simulink model "BionicBaroreflex"  (Simulink 7.5)
settings: Solver=ode45  StartTime=0.0  StopTime=3600  RelTol=1e-3
undefined symbols (not defined in the file or in its folder): get
libraries: simulink x11, dspstat3 x4, dspsnks4 x2, dspbuff3 x2, dspspect3 x2
settings Model: Creator=admin  LastModifiedBy=Peidro
settings DebuggingCC: StrictBusMsg=Warning

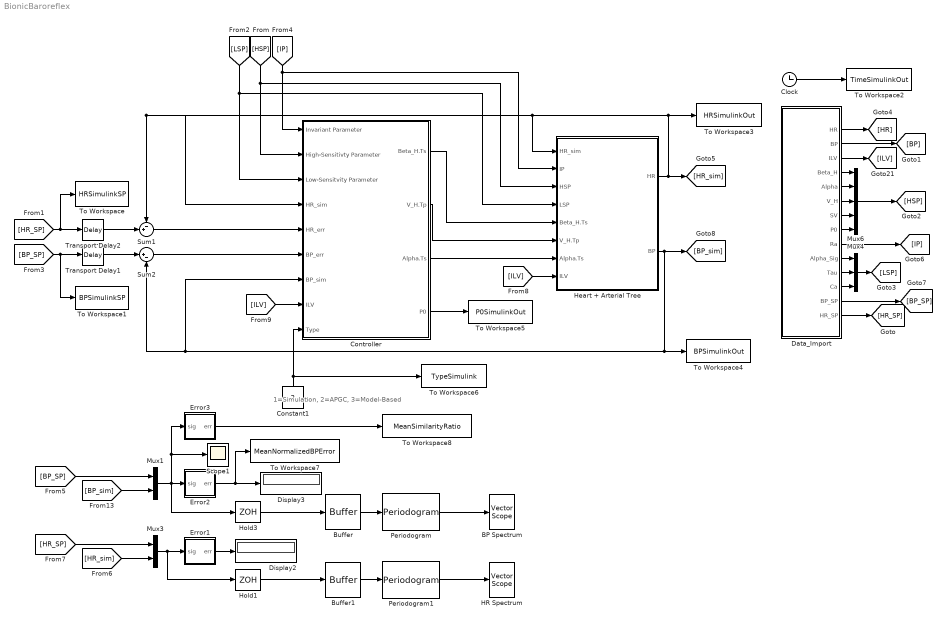
== system BionicBaroreflex ==
  note: 1=Simulation,
      | 2=APGC,
      | 3=Model-Based
  BP Spectrum : dspsnks4/Vector Scope  DialogController=dspdialog.VectorScope  DialogControllerArgs=DataTag0  ScopeProperties=on  Domain=Frequency  HorizSpan=1  DisplayProperties=off  AxisGrid=on  Memory=on  FrameNumber=on  AxisLegend=on  AxisZoom=off  OpenScopeAtSimStart=on  OpenScopeImmediately=off  FigPos=get(0,'defaultfigureposition')  AxisProperties=off  XUnits=Hertz  XRange=[0...Fs/2]  InheritXIncr=off  XIncr=1  XLabel=Time  XLimit=Auto  XMin=0  XMax=0.5  XStart=0  YUnits=dB  YLabel=Amplitude  LineProperties=off  LineColors=[1 0 0]|[0 0 1]  XAxisParamsVer=6.9
      settings: YMin=-106.7264  YMax=8.3849
  Buffer : dspbuff3/Buffer  N=128  V=64  ic=0
  Buffer1 : dspbuff3/Buffer  N=128  V=64  ic=0
  Clock : Clock
      settings: Decimation=10
  Constant1 : Constant  Value=2  OutDataType=fixdt(1, 16)  OutScaling=2^0
  Controller : Subsystem
  Data_Import : Subsystem
  Display2 : Display
  Display3 : Display
  Error1 : Subsystem
  Error2 : Subsystem
  Error3 : Subsystem
  HR Spectrum : dspsnks4/Vector Scope  DialogController=dspdialog.VectorScope  DialogControllerArgs=DataTag5  ScopeProperties=on  Domain=Frequency  HorizSpan=1  DisplayProperties=off  AxisGrid=on  Memory=on  FrameNumber=on  AxisLegend=on  AxisZoom=off  OpenScopeAtSimStart=on  OpenScopeImmediately=off  FigPos=get(0,'defaultfigureposition')  AxisProperties=off  XUnits=Hertz  XRange=[0...Fs/2]  InheritXIncr=off  XIncr=1  XLabel=Time  XLimit=Auto  XMin=0  XMax=0.5  XStart=0  YUnits=dB  YLabel=Amplitude  LineProperties=off  LineColors=[1 0 0]|[0 0 1]  XAxisParamsVer=6.9
      settings: YMin=-106.7264  YMax=8.3849
  Heart + Arterial Tree : Subsystem
  Hold1 : ZeroOrderHold  SampleTime=10
  Hold3 : ZeroOrderHold  SampleTime=10
  Mux1 : Mux  Inputs=2
  Mux3 : Mux  Inputs=2
  Mux4 : Mux  Inputs=3
  Mux6 : Mux  Inputs=5
  Periodogram : dspspect3/Periodogram  SystemSampleTime=-1  measurement=Power spectral density  wintype=Hamming  Rs=50  beta=5  winsamp=Periodic  inheritFFT=off  fftsize=128  navg=2  inheritTs=on  Ts=1
  Periodogram1 : dspspect3/Periodogram  SystemSampleTime=-1  measurement=Power spectral density  wintype=Hamming  Rs=50  beta=5  winsamp=Periodic  inheritFFT=off  fftsize=128  navg=2  inheritTs=on  Ts=1
  Scope1 : Scope
      settings: YMin=67.5  YMax=125
  Sum1 : Sum  Inputs=-+|  OutDataType=fixdt(1, 16)  OutScaling=2^0
  Sum2 : Sum  Inputs=|+-  OutDataType=fixdt(1, 16)  OutScaling=2^0
  To Workspace : ToWorkspace  VariableName=HRSimulinkSP  SampleTime=-1  SaveFormat=Structure
  To Workspace1 : ToWorkspace  VariableName=BPSimulinkSP  SampleTime=-1  SaveFormat=Structure
  To Workspace2 : ToWorkspace  VariableName=TimeSimulinkOut  SampleTime=-1  SaveFormat=Structure
  To Workspace3 : ToWorkspace  VariableName=HRSimulinkOut  SampleTime=-1  SaveFormat=Structure
  To Workspace4 : ToWorkspace  VariableName=BPSimulinkOut  SampleTime=-1  SaveFormat=Structure
  To Workspace5 : ToWorkspace  VariableName=P0SimulinkOut  SampleTime=-1  SaveFormat=Structure
  To Workspace6 : ToWorkspace  VariableName=TypeSimulink  SampleTime=-1  SaveFormat=Structure
  To Workspace7 : ToWorkspace  VariableName=MeanNormalizedBPError  SampleTime=-1  SaveFormat=Structure
  To Workspace8 : ToWorkspace  VariableName=MeanSimilarityRatio  SampleTime=-1  SaveFormat=Structure
  Transport Delay1 : TransportDelay  DelayTime=10
  Transport Delay2 : TransportDelay  DelayTime=10
  wires:
  Data_Import/1(HR) -> [HR]
  [ILV] -> Controller/8(ILV)
  Heart + Arterial Tree/1(HR) -> [HR_sim], To Workspace3/1, Sum1/1, Controller/4(HR_sim), Heart + Arterial Tree/1(HR_sim)
  Controller/1(Beta_H.Ts) -> Heart + Arterial Tree/5(Beta_H.Ts)
  Controller/2(V_H.Tp) -> Heart + Arterial Tree/6(V_H.Tp)
  Controller/3(Alpha.Ts) -> Heart + Arterial Tree/7(Alpha.Ts)
  Constant1/1 -> Controller/9(Type), To Workspace6/1
  Heart + Arterial Tree/2(BP) -> [BP_sim], Sum2/2, Controller/7(BP_sim), To Workspace4/1
  [BP_SP] -> To Workspace1/1, Transport Delay1/1
  [HR_SP] -> To Workspace/1, Transport Delay2/1
  [HSP] -> Controller/2(High-Sensitivty Parameter), Heart + Arterial Tree/3(HSP)
  [LSP] -> Controller/3(Low-Sensitvity Parameter), Heart + Arterial Tree/4(LSP)
  Mux6/1 -> [HSP]
  Mux4/1 -> [LSP]
  [IP] -> Controller/1(Invariant Parameter), Heart + Arterial Tree/2(IP)
  Mux1/1 -> Error2/1(sig), Hold3/1, Scope1/1, Error3/1(sig)
  Error2/1(err) -> Display3/1, To Workspace7/1
  Mux3/1 -> Error1/1(sig), Hold1/1
  Error1/1(err) -> Display2/1
  [HR_SP] -> Mux3/1
  [HR_sim] -> Mux3/2
  [BP_SP] -> Mux1/1
  Sum1/1 -> Controller/5(HR_err)
  Sum2/1 -> Controller/6(BP_err)
  Periodogram/1 -> BP Spectrum/1
  Hold3/1 -> Buffer/1
  Buffer/1 -> Periodogram/1
  [BP_sim] -> Mux1/2
  Periodogram1/1 -> HR Spectrum/1
  Hold1/1 -> Buffer1/1
  Buffer1/1 -> Periodogram1/1
  Data_Import/2(BP) -> [BP]
  Data_Import/3(ILV) -> [ILV]
  Data_Import/4(Beta_H) -> Mux6/1
  Data_Import/5(Alpha) -> Mux6/2
  Data_Import/6(V_H) -> Mux6/3
  Data_Import/7(SV) -> Mux6/4
  Data_Import/8(P0) -> Mux6/5
  Data_Import/9(Ra) -> [IP]
  Data_Import/10(Alpha_Sig) -> Mux4/1
  Data_Import/11(Tau) -> Mux4/2
  Data_Import/12(Ca) -> Mux4/3
  Data_Import/13(BP_SP) -> [BP_SP]
  Data_Import/14(HR_SP) -> [HR_SP]
  Clock/1 -> To Workspace2/1
  Controller/4(P0) -> To Workspace5/1
  [ILV] -> Heart + Arterial Tree/8(ILV)
  Transport Delay2/1 -> Sum1/2
  Transport Delay1/1 -> Sum2/1
  Error3/1(err) -> To Workspace8/1

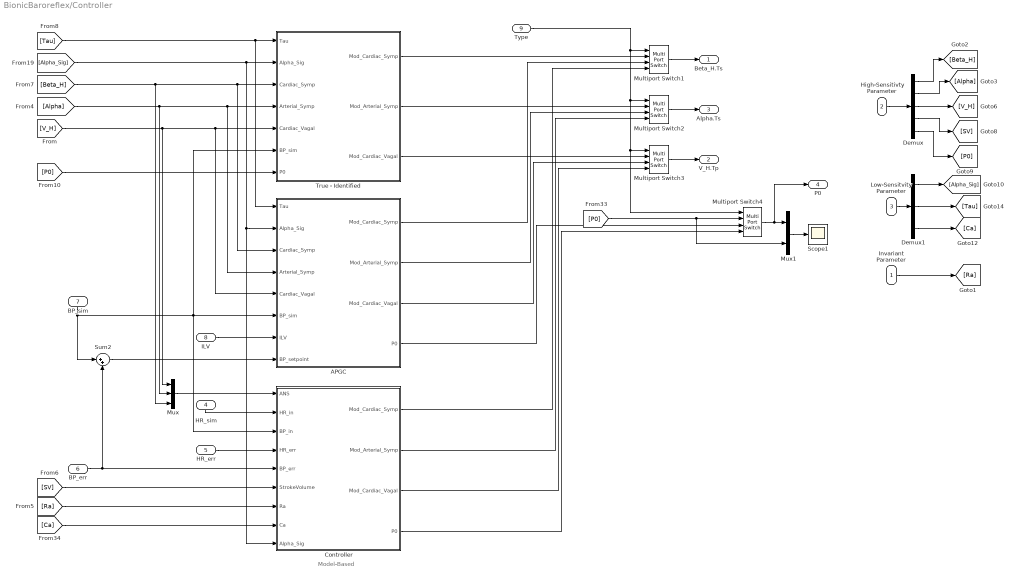
== system BionicBaroreflex/Controller ==
  note: Model-Based
  Invariant Parameter : Inport
  High-Sensitivty Parameter : Inport  Port=2
  Low-Sensitvity Parameter : Inport  Port=3
  HR_sim : Inport  Port=4
  HR_err : Inport  Port=5
  BP_err : Inport  Port=6
  BP_sim : Inport  Port=7
  ILV : Inport  Port=8
  Type : Inport  Port=9
  "APGC " : Subsystem
  Controller : Subsystem
  Demux : Demux  Outputs=5
  Demux1 : Demux  Outputs=3
  Multiport Switch{1..4} (4 alike) : MultiPortSwitch  zeroidx=off  OutDataType=fixdt(1, 16)  OutScaling=2^0
  Mux : Mux  Inputs=3
  Mux1 : Mux  Inputs=2
  Scope1 : Scope
      settings: YMin=1.725  YMax=1.925  SaveName=ScopeData2
  Sum2 : Sum  Inputs=|++  OutDataType=fixdt(1, 16)  OutScaling=2^0
  True - Identified : Subsystem
  Beta_H.Ts : Outport
  V_H.Tp : Outport  Port=2
  Alpha.Ts : Outport  Port=3
  P0 : Outport  Port=4
  wires:
  [Tau] -> True - Identified/1(Tau), "APGC "/1(Tau)
  [Beta_H] -> True - Identified/3(Cardiac_Symp), "APGC "/3(Cardiac_Symp), Mux/3
  [Alpha] -> True - Identified/4(Arterial_Symp), "APGC "/4(Arterial_Symp), Mux/2
  [V_H] -> True - Identified/5(Cardiac_Vagal), "APGC "/5(Cardiac_Vagal), Mux/1
  BP_sim/1 -> True - Identified/6(BP_sim), Controller/3(BP_in), "APGC "/6(BP_sim), Sum2/1
  [P0] -> True - Identified/7(P0)
  ILV/1 -> "APGC "/7(ILV)
  True - Identified/1(Mod_Cardiac_Symp) -> Multiport Switch1/2
  Multiport Switch1/1 -> Beta_H.Ts/1
  True - Identified/2(Mod_Arterial_Symp) -> Multiport Switch2/2
  True - Identified/3(Mod_Cardiac_Vagal) -> Multiport Switch3/2
  Controller/1(Mod_Cardiac_Symp) -> Multiport Switch1/4
  Controller/2(Mod_Arterial_Symp) -> Multiport Switch2/4
  Controller/3(Mod_Cardiac_Vagal) -> Multiport Switch3/4
  Mux/1 -> Controller/1(ANS)
  Type/1 -> Multiport Switch2/1, Multiport Switch3/1, Multiport Switch4/1, Multiport Switch1/1
  Controller/4(P0) -> Multiport Switch4/4
  [Ra] -> Controller/7(Ra)
  [Ca] -> Controller/8(Ca)
  [SV] -> Controller/6(StrokeVolume)
  HR_err/1 -> Controller/4(HR_err)
  BP_err/1 -> Sum2/2, Controller/5(BP_err)
  High-Sensitivty Parameter/1 -> Demux/1
  Demux/1 -> [Beta_H]
  Demux/2 -> [Alpha]
  Demux/3 -> [V_H]
  Demux/4 -> [SV]
  Demux/5 -> [P0]
  Low-Sensitvity Parameter/1 -> Demux1/1
  Demux1/1 -> [Alpha_Sig]
  Demux1/2 -> [Tau]
  Demux1/3 -> [Ca]
  [Alpha_Sig] -> True - Identified/2(Alpha_Sig), "APGC "/2(Alpha_Sig), Controller/9(Alpha_Sig)
  Invariant Parameter/1 -> [Ra]
  HR_sim/1 -> Controller/2(HR_in)
  Multiport Switch2/1 -> Alpha.Ts/1
  Multiport Switch3/1 -> V_H.Tp/1
  Sum2/1 -> "APGC "/8(BP_setpoint)
  [P0] -> Multiport Switch4/2, Mux1/2
  Multiport Switch4/1 -> Mux1/1, P0/1
  Mux1/1 -> Scope1/1
  "APGC "/1(Mod_Cardiac_Symp) -> Multiport Switch1/3
  "APGC "/2(Mod_Arterial_Symp) -> Multiport Switch2/3
  "APGC "/3(Mod_Cardiac_Vagal) -> Multiport Switch3/3
  "APGC "/4(P0) -> Multiport Switch4/3

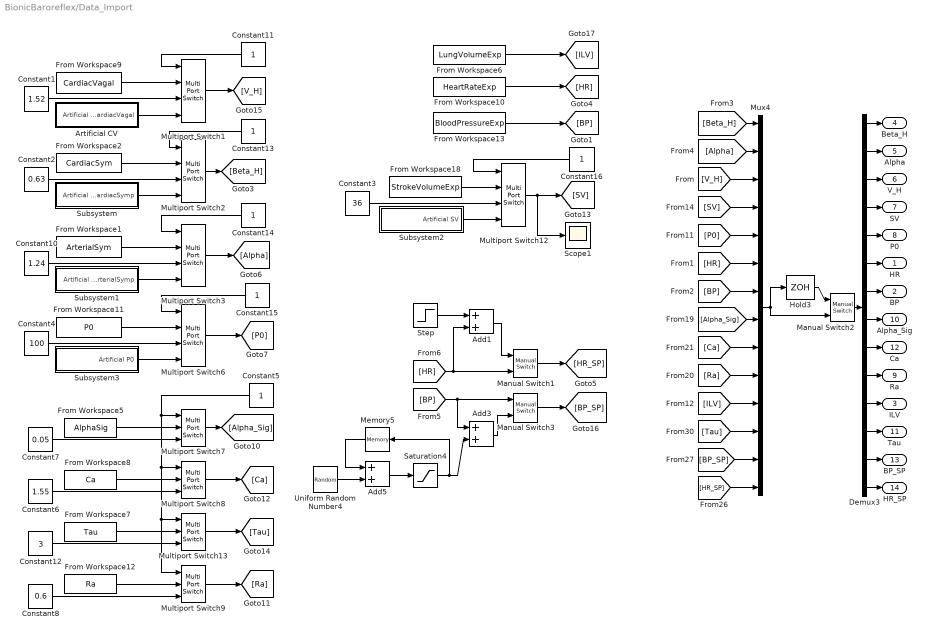
== system BionicBaroreflex/Data_Import ==
  Add1 : Sum  OutDataType=fixdt(1, 16)  OutScaling=2^-10
  Add3 : Sum  OutDataType=fixdt(1, 16)  OutScaling=2^-10
  Add5 : Sum  OutDataType=fixdt(1, 16)  OutScaling=2^-10
  Artificial CV : Subsystem
  Constant1 : Constant  Value=1.52  OutDataType=fixdt(1, 16)  OutScaling=2^0
  Constant10 : Constant  Value=1.24  OutDataType=fixdt(1, 16)  OutScaling=2^0
  Constant{5,11,13..16} (6 alike) : Constant  OutDataType=fixdt(1, 16)  OutScaling=2^0
  Constant12 : Constant  Value=3  OutDataType=fixdt(1, 16)  OutScaling=2^0
  Constant2 : Constant  Value=0.63  OutDataType=fixdt(1, 16)  OutScaling=2^0
  Constant3 : Constant  Value=36  OutDataType=fixdt(1, 16)  OutScaling=2^0
  Constant4 : Constant  Value=100  OutDataType=fixdt(1, 16)  OutScaling=2^0
  Constant6 : Constant  Value=1.55  OutDataType=fixdt(1, 16)  OutScaling=2^0
  Constant7 : Constant  Value=0.05  OutDataType=fixdt(1, 16)  OutScaling=2^0
  Constant8 : Constant  Value=0.6  OutDataType=fixdt(1, 16)  OutScaling=2^0
  Demux3 : Demux  Outputs=14
  From Workspace1 : FromWorkspace  VariableName=ArterialSym  SampleTime=1
  From Workspace10 : FromWorkspace  VariableName=HeartRateExp  SampleTime=1
  From Workspace11 : FromWorkspace  VariableName=P0  SampleTime=1
  From Workspace12 : FromWorkspace  VariableName=Ra  SampleTime=0
  From Workspace13 : FromWorkspace  VariableName=BloodPressureExp  SampleTime=1
  From Workspace18 : FromWorkspace  VariableName=StrokeVolumeExp  SampleTime=1
  From Workspace2 : FromWorkspace  VariableName=CardiacSym  SampleTime=1
  From Workspace5 : FromWorkspace  VariableName=AlphaSig  SampleTime=0
  From Workspace6 : FromWorkspace  VariableName=LungVolumeExp  SampleTime=1
  From Workspace7 : FromWorkspace  VariableName=Tau  SampleTime=0
  From Workspace8 : FromWorkspace  VariableName=Ca  SampleTime=0
  From Workspace9 : FromWorkspace  VariableName=CardiacVagal  SampleTime=1
  Hold3 : ZeroOrderHold  SampleTime=5
  Manual Switch1 : simulink/Signal Routing/Manual Switch  SystemSampleTime=-1  sw=0  action=0  varsize=off
  Manual Switch2 : simulink/Signal Routing/Manual Switch  SystemSampleTime=-1  sw=0  action=0  varsize=off
  Manual Switch3 : simulink/Signal Routing/Manual Switch  SystemSampleTime=-1  sw=1  action=0  varsize=off
  Memory5 : Memory  X0=1.3
  Multiport Switch{1..3,6,12} (5 alike) : MultiPortSwitch  zeroidx=off  OutDataType=fixdt(1, 16)  OutScaling=2^0
  Multiport Switch{7..9,13} (4 alike) : MultiPortSwitch  Inputs=2  zeroidx=off  OutDataType=fixdt(1, 16)  OutScaling=2^0
  Mux4 : Mux  Inputs=14
  Saturation4 : Saturate  UpperLimit=25  LowerLimit=-25  OutDataType=fixdt(1, 16)  OutScaling=2^0
  Scope1 : Scope
      settings: YMin=1  YMax=1.95  SaveName=ScopeData5
  Step : Step  Time=1000  SampleTime=0
  Subsystem : Subsystem
  Subsystem1 : Subsystem
  Subsystem2 : Subsystem
  Subsystem3 : Subsystem
  Uniform Random Number4 : UniformRandomNumber  Minimum=-0.1  Maximum=0.1  SampleTime=500
  HR : Outport
  BP : Outport  Port=2
  ILV : Outport  Port=3
  Beta_H : Outport  Port=4
  Alpha : Outport  Port=5
  V_H : Outport  Port=6
  SV : Outport  Port=7
  P0 : Outport  Port=8
  Ra : Outport  Port=9
  Alpha_Sig : Outport  Port=10
  Tau : Outport  Port=11
  Ca : Outport  Port=12
  BP_SP : Outport  Port=13
  HR_SP : Outport  Port=14
  wires:
  [V_H] -> Mux4/3
  [SV] -> Mux4/4
  [Alpha] -> Mux4/2
  [P0] -> Mux4/5
  [Beta_H] -> Mux4/1
  Hold3/1 -> Manual Switch2/1
  Manual Switch2/1 -> Demux3/1
  Demux3/1 -> Beta_H/1
  Demux3/3 -> V_H/1
  Demux3/2 -> Alpha/1
  Demux3/4 -> SV/1
  Demux3/5 -> P0/1
  [HR] -> Mux4/6
  [BP] -> Mux4/7
  Demux3/6 -> HR/1
  Demux3/7 -> BP/1
  [Alpha_Sig] -> Mux4/8
  Demux3/8 -> Alpha_Sig/1
  Mux4/1 -> Hold3/1, Manual Switch2/2
  [Ca] -> Mux4/9
  [Ra] -> Mux4/10
  Demux3/9 -> Ca/1
  Demux3/10 -> Ra/1
  From Workspace5/1 -> Multiport Switch7/2
  From Workspace8/1 -> Multiport Switch8/2
  From Workspace12/1 -> Multiport Switch9/2
  Multiport Switch7/1 -> [Alpha_Sig]
  Multiport Switch8/1 -> [Ca]
  Multiport Switch9/1 -> [Ra]
  Constant6/1 -> Multiport Switch8/3
  Constant7/1 -> Multiport Switch7/3
  Constant8/1 -> Multiport Switch9/3
  Constant5/1 -> Multiport Switch7/1, Multiport Switch8/1, Multiport Switch13/1, Multiport Switch9/1
  [ILV] -> Mux4/11
  Demux3/11 -> ILV/1
  From Workspace7/1 -> Multiport Switch13/2
  Multiport Switch13/1 -> [Tau]
  Constant12/1 -> Multiport Switch13/3
  [Tau] -> Mux4/12
  Demux3/12 -> Tau/1
  From Workspace10/1 -> [HR]
  From Workspace13/1 -> [BP]
  Demux3/13 -> BP_SP/1
  Demux3/14 -> HR_SP/1
  [HR_SP] -> Mux4/14
  [BP_SP] -> Mux4/13
  From Workspace6/1 -> [ILV]
  From Workspace18/1 -> Multiport Switch12/2
  Constant3/1 -> Multiport Switch12/3
  Constant16/1 -> Multiport Switch12/1
  Multiport Switch12/1 -> [SV], Scope1/1
  Multiport Switch6/1 -> [P0]
  Multiport Switch3/1 -> [Alpha]
  Multiport Switch2/1 -> [Beta_H]
  Multiport Switch1/1 -> [V_H]
  From Workspace9/1 -> Multiport Switch1/2
  From Workspace2/1 -> Multiport Switch2/2
  From Workspace1/1 -> Multiport Switch3/2
  From Workspace11/1 -> Multiport Switch6/2
  Constant1/1 -> Multiport Switch1/3
  Constant2/1 -> Multiport Switch2/3
  Constant10/1 -> Multiport Switch3/3
  Constant4/1 -> Multiport Switch6/3
  Constant11/1 -> Multiport Switch1/1
  Constant13/1 -> Multiport Switch2/1
  Constant14/1 -> Multiport Switch3/1
  Constant15/1 -> Multiport Switch6/1
  Artificial CV/1(Artificial CardiacVagal) -> Multiport Switch1/4
  Subsystem/1(Artificial CardiacSymp) -> Multiport Switch2/4
  Subsystem1/1(Artificial ArterialSymp) -> Multiport Switch3/4
  Subsystem3/1(Artificial P0) -> Multiport Switch6/4
  Subsystem2/1(Artificial SV) -> Multiport Switch12/4
  [HR] -> Manual Switch1/2, Add1/2
  Manual Switch1/1 -> [HR_SP]
  [BP] -> Manual Switch3/1, Add3/1
  Manual Switch3/1 -> [BP_SP]
  Step/1 -> Add1/1
  Add1/1 -> Manual Switch1/1
  Memory5/1 -> Add5/1
  Uniform Random Number4/1 -> Add5/2
  Add5/1 -> Saturation4/1
  Saturation4/1 -> Memory5/1, Add3/2
  Add3/1 -> Manual Switch3/2

== system BionicBaroreflex/Error1 ==
  sig : Inport
  Abs1 : Abs  OutDataType=fixdt(1, 16)  OutScaling=2^0
  Add1 : Sum  Inputs=-+  OutDataType=fixdt(1, 16)  OutScaling=2^-10
  Correlation : dspstat3/Correlation  DialogController=dspDDGCreate  DialogControllerArgs=DataTag1  domain=Time  outputDataTypeStr=Inherit: Same as accumulator  outputLastDataTypeStr=Inherit: Same as accumulator  outputMin=[]  outputMax=[]  roundingMode=Floor  overflowMode=off
  Demux : Demux  Outputs=2
  Divide : Product  Inputs=/*  OutDataType=fixdt(1, 16)  OutScaling=2^-10
  Mean : dspstat3/Mean  DialogController=dspDDGCreate  DialogControllerArgs=DataTag2  run=off  reset_popup=None  directionMode=Each column  dimension=1  treatSBRowAsCol=on  roiEnable=off  roiType=Rectangles  roiPortion=Entire ROI  roiOutput=Individual statistics for each ROI  roiFlag=off  outputDataTypeStr=Inherit: Same as accumulator  outputLastDataTypeStr=Inherit: Same as accumulator  outputMin=[]  outputMax=[]  roundingMode=Floor  overflowMode=off
  Scope : Scope
      settings: SaveName=ScopeData4
  err : Outport
  wires:
  sig/1 -> Demux/1
  Mean/1 -> err/1
  Divide/1 -> Mean/1
  Abs1/1 -> Divide/2
  Demux/2 -> Add1/2, Correlation/2
  Demux/1 -> Divide/1, Add1/1, Correlation/1
  Add1/1 -> Abs1/1
  Correlation/1 -> Scope/1

== system BionicBaroreflex/Error2 ==
  sig : Inport
  Abs1 : Abs  OutDataType=fixdt(1, 16)  OutScaling=2^0
  Add1 : Sum  Inputs=-+  OutDataType=fixdt(1, 16)  OutScaling=2^-10
  Demux : Demux  Outputs=2
  Divide : Product  Inputs=/*  OutDataType=fixdt(1, 16)  OutScaling=2^-10
  Mean : dspstat3/Mean  DialogController=dspDDGCreate  DialogControllerArgs=DataTag3  run=off  reset_popup=None  directionMode=Each column  dimension=1  treatSBRowAsCol=on  roiEnable=off  roiType=Rectangles  roiPortion=Entire ROI  roiOutput=Individual statistics for each ROI  roiFlag=off  outputDataTypeStr=Inherit: Same as accumulator  outputLastDataTypeStr=Inherit: Same as accumulator  outputMin=[]  outputMax=[]  roundingMode=Floor  overflowMode=off
  err : Outport
  wires:
  Add1/1 -> Abs1/1
  Demux/1 -> Add1/1, Divide/1
  Demux/2 -> Add1/2
  Abs1/1 -> Divide/2
  Divide/1 -> Mean/1
  Mean/1 -> err/1
  sig/1 -> Demux/1

== system BionicBaroreflex/Error3 ==
  sig : Inport
  Demux : Demux  Outputs=2
  Divide : Product  Inputs=/*  OutDataType=fixdt(1, 16)  OutScaling=2^-10
  Mean : dspstat3/Mean  DialogController=dspDDGCreate  DialogControllerArgs=DataTag4  run=off  reset_popup=None  directionMode=Each column  dimension=1  treatSBRowAsCol=on  roiEnable=off  roiType=Rectangles  roiPortion=Entire ROI  roiOutput=Individual statistics for each ROI  roiFlag=off  outputDataTypeStr=Inherit: Same as accumulator  outputLastDataTypeStr=Inherit: Same as accumulator  outputMin=[]  outputMax=[]  roundingMode=Floor  overflowMode=off
  err : Outport
  wires:
  sig/1 -> Demux/1
  Mean/1 -> err/1
  Divide/1 -> Mean/1
  Demux/2 -> Divide/2
  Demux/1 -> Divide/1

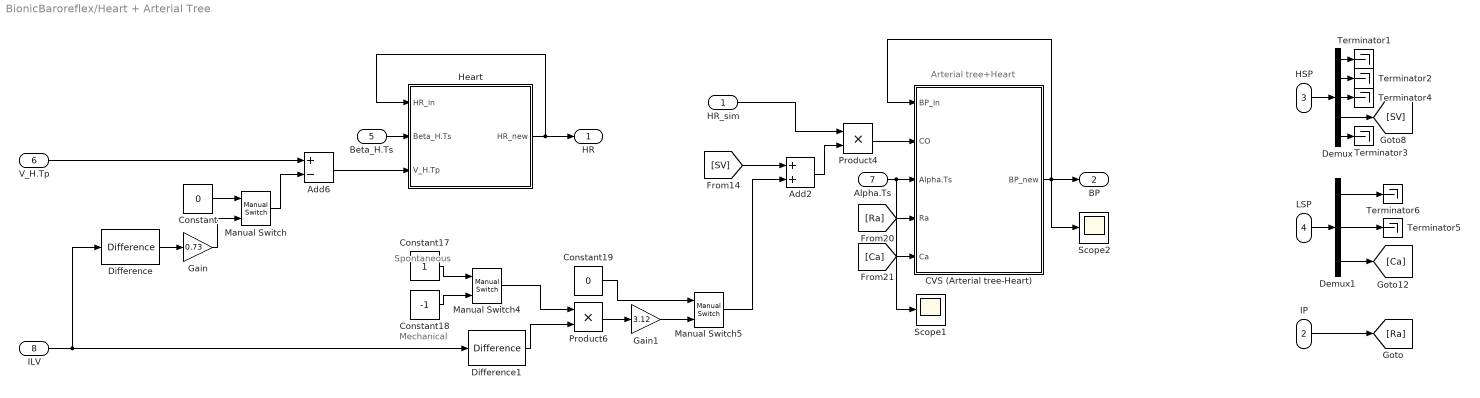
== system BionicBaroreflex/Heart + Arterial Tree ==
  note: Arterial tree+Heart
  note: Mechanical
  note: Spontaneous
  HR_sim : Inport
  IP : Inport  Port=2
  HSP : Inport  Port=3
  LSP : Inport  Port=4
  Beta_H.Ts : Inport  Port=5
  V_H.Tp : Inport  Port=6
  Alpha.Ts : Inport  Port=7
  ILV : Inport  Port=8
  Add2 : Sum  OutDataType=fixdt(1, 16)  OutScaling=2^-10
  Add6 : Sum  Inputs=+-  OutDataType=fixdt(1, 16)  OutScaling=2^-10
  CVS (Arterial tree-Heart) : Subsystem
  Constant : Constant  Value=0  OutDataType=fixdt(1, 16)  OutScaling=2^0
  Constant17 : Constant  OutDataType=fixdt(1, 16)  OutScaling=2^0
  Constant18 : Constant  Value=-1  OutDataType=fixdt(1, 16)  OutScaling=2^0
  Constant19 : Constant  Value=0  OutDataType=fixdt(1, 16)  OutScaling=2^0
  Demux : Demux  Outputs=5
  Demux1 : Demux  Outputs=3
  Difference : simulink/Discrete/Difference  SystemSampleTime=-1  ICPrevInput=0.0  OutMin=[]  OutMax=[]  OutDataType=fixdt(1, 16)  OutScaling=2^-10  DoSatur=off
  Difference1 : simulink/Discrete/Difference  SystemSampleTime=-1  ICPrevInput=0.0  OutMin=[]  OutMax=[]  OutDataType=fixdt(1, 16)  OutScaling=2^-10  DoSatur=off
  Gain : Gain  Gain=0.73  ParameterDataType=fixdt(1, 16)  ParameterScaling=2^0  OutDataType=fixdt(1, 16)  OutScaling=2^0
  Gain1 : Gain  Gain=3.12  ParameterDataType=fixdt(1, 16)  ParameterScaling=2^0  OutDataType=fixdt(1, 16)  OutScaling=2^0
  Heart : Subsystem
  Manual Switch : simulink/Signal Routing/Manual Switch  SystemSampleTime=-1  sw=1  action=0  varsize=off
  Manual Switch4 : simulink/Signal Routing/Manual Switch  SystemSampleTime=-1  sw=1  action=0  varsize=off
  Manual Switch5 : simulink/Signal Routing/Manual Switch  SystemSampleTime=-1  sw=1  action=0  varsize=off
  Product4 : Product  OutDataType=fixdt(1, 16)  OutScaling=2^0  RndMeth=Zero
  Product6 : Product  OutDataType=fixdt(1, 16)  OutScaling=2^0  RndMeth=Zero
  Scope1 : Scope
      settings: YMin=-1500  YMax=1250  SaveName=ScopeData11
  Scope2 : Scope
      settings: YMin=-1500  YMax=1250
  Terminator{1..6} (6 alike) : Terminator
  HR : Outport
  BP : Outport  Port=2
  wires:
  CVS (Arterial tree-Heart)/1(BP_new) -> CVS (Arterial tree-Heart)/1(BP_in), BP/1, Scope2/1
  Heart/1(HR_new) -> Heart/1(HR_in), HR/1
  [Ra] -> CVS (Arterial tree-Heart)/4(Ra)
  [Ca] -> CVS (Arterial tree-Heart)/5(Ca)
  Beta_H.Ts/1 -> Heart/2(Beta_H.Ts)
  Alpha.Ts/1 -> CVS (Arterial tree-Heart)/3(Alpha.Ts), Scope1/1
  LSP/1 -> Demux1/1
  Demux1/1 -> Terminator6/1
  Demux1/2 -> Terminator5/1
  Demux1/3 -> [Ca]
  IP/1 -> [Ra]
  HSP/1 -> Demux/1
  Demux/1 -> Terminator1/1
  Demux/2 -> Terminator2/1
  Demux/3 -> Terminator4/1
  Demux/4 -> [SV]
  Demux/5 -> Terminator3/1
  Product4/1 -> CVS (Arterial tree-Heart)/2(CO)
  Constant17/1 -> Manual Switch4/1
  Constant18/1 -> Manual Switch4/2
  Manual Switch4/1 -> Product6/1
  Difference1/1 -> Product6/2
  Product6/1 -> Gain1/1
  Manual Switch5/1 -> Add2/2
  Constant19/1 -> Manual Switch5/1
  ILV/1 -> Difference1/1, Difference/1
  Gain1/1 -> Manual Switch5/2
  HR_sim/1 -> Product4/1
  [SV] -> Add2/1
  Add2/1 -> Product4/2
  Gain/1 -> Manual Switch/2
  Constant/1 -> Manual Switch/1
  Difference/1 -> Gain/1
  Add6/1 -> Heart/3(V_H.Tp)
  V_H.Tp/1 -> Add6/1
  Manual Switch/1 -> Add6/2

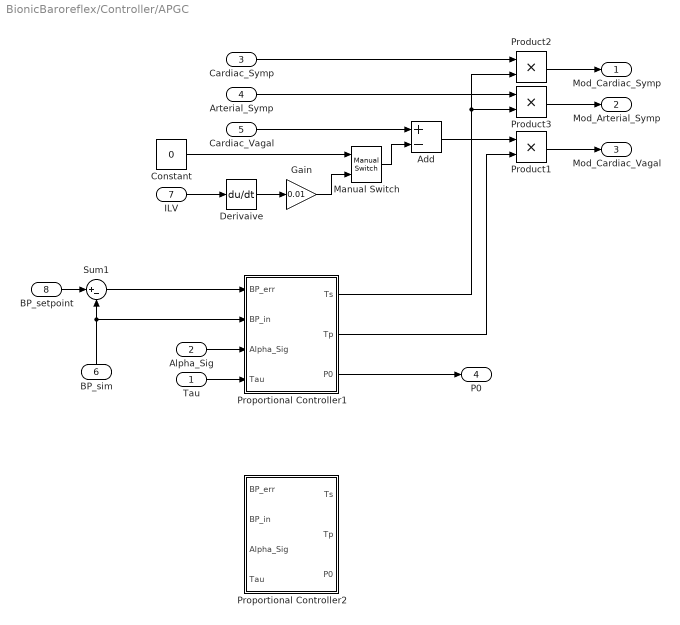
== system BionicBaroreflex/Controller/APGC  ==
  Tau : Inport
  Alpha_Sig : Inport  Port=2
  Cardiac_Symp : Inport  Port=3
  Arterial_Symp : Inport  Port=4
  Cardiac_Vagal : Inport  Port=5
  BP_sim : Inport  Port=6
  ILV : Inport  Port=7
  BP_setpoint : Inport  Port=8
  Add : Sum  Inputs=+-  OutDataType=fixdt(1, 16)  OutScaling=2^-10
  Constant : Constant  Value=0  OutDataType=fixdt(1, 16)  OutScaling=2^0
  Derivaive : Derivative
  Gain : Gain  Gain=0.01  ParameterDataType=fixdt(1, 16)  ParameterScaling=2^0  OutDataType=fixdt(1, 16)  OutScaling=2^0
  Manual Switch : simulink/Signal Routing/Manual Switch  SystemSampleTime=-1  sw=1  action=0  varsize=off
  Product1 : Product  OutDataType=fixdt(1, 16)  OutScaling=2^0  RndMeth=Zero
  Product2 : Product  OutDataType=fixdt(1, 16)  OutScaling=2^0  RndMeth=Zero
  Product3 : Product  OutDataType=fixdt(1, 16)  OutScaling=2^0  RndMeth=Zero
  Proportional Controller1 : Subsystem
  Proportional Controller2 : Subsystem
  Sum1 : Sum  Inputs=|+-  OutDataType=fixdt(1, 16)  OutScaling=2^0
  Mod_Cardiac_Symp : Outport
  Mod_Arterial_Symp : Outport  Port=2
  Mod_Cardiac_Vagal : Outport  Port=3
  P0 : Outport  Port=4
  wires:
  Cardiac_Symp/1 -> Product2/1
  Product2/1 -> Mod_Cardiac_Symp/1
  Arterial_Symp/1 -> Product3/1
  Product3/1 -> Mod_Arterial_Symp/1
  Product1/1 -> Mod_Cardiac_Vagal/1
  Add/1 -> Product1/1
  Cardiac_Vagal/1 -> Add/1
  ILV/1 -> Derivaive/1
  Derivaive/1 -> Gain/1
  Gain/1 -> Manual Switch/2
  Manual Switch/1 -> Add/2
  Constant/1 -> Manual Switch/1
  Proportional Controller1/3(P0) -> P0/1
  Proportional Controller1/2(Tp) -> Product1/2
  Proportional Controller1/1(Ts) -> Product3/2, Product2/2
  BP_setpoint/1 -> Sum1/1
  Sum1/1 -> Proportional Controller1/1(BP_err)
  Alpha_Sig/1 -> Proportional Controller1/3(Alpha_Sig)
  Tau/1 -> Proportional Controller1/4(Tau)
  BP_sim/1 -> Sum1/2, Proportional Controller1/2(BP_in)

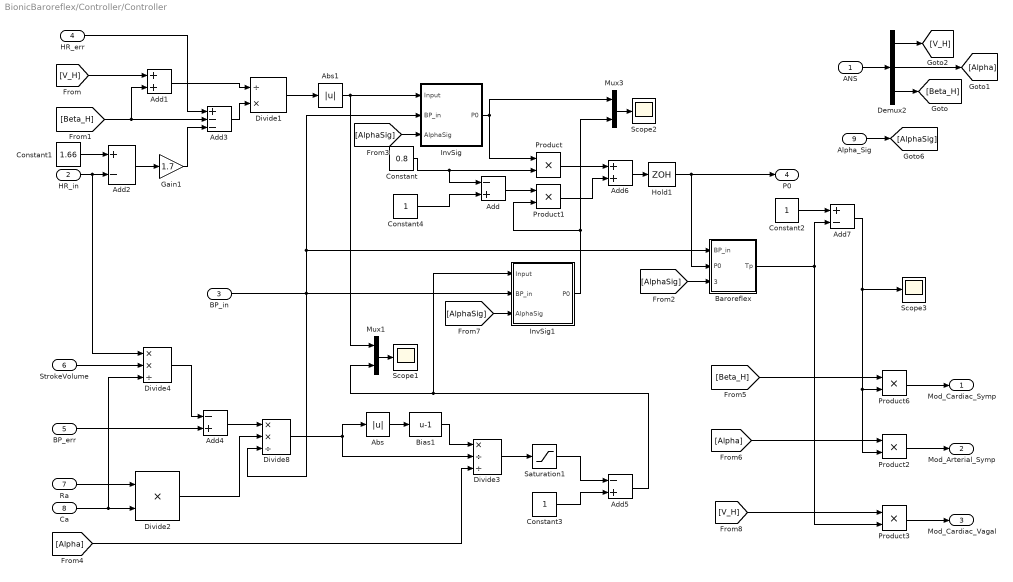
== system BionicBaroreflex/Controller/Controller ==
  ANS : Inport
  HR_in : Inport  Port=2
  BP_in : Inport  Port=3
  HR_err : Inport  Port=4
  BP_err : Inport  Port=5
  StrokeVolume : Inport  Port=6
  Ra : Inport  Port=7
  Ca : Inport  Port=8
  Alpha_Sig : Inport  Port=9
  Abs : Abs  OutDataType=fixdt(1, 16)  OutScaling=2^0
  Abs1 : Abs  OutDataType=fixdt(1, 16)  OutScaling=2^0
  Add : Sum  Inputs=-+  OutDataType=fixdt(1, 16)  OutScaling=2^-10
  Add1 : Sum  OutDataType=fixdt(1, 16)  OutScaling=2^-10
  Add2 : Sum  Inputs=+-  OutDataType=fixdt(1, 16)  OutScaling=2^-10
  Add3 : Sum  Inputs=+--  OutDataType=fixdt(1, 16)  OutScaling=2^-10
  Add4 : Sum  Inputs=-+  OutDataType=fixdt(1, 16)  OutScaling=2^-10
  Add5 : Sum  Inputs=-+  OutDataType=fixdt(1, 16)  OutScaling=2^-10
  Add6 : Sum  OutDataType=fixdt(1, 16)  OutScaling=2^-10
  Add7 : Sum  Inputs=+-  OutDataType=fixdt(1, 16)  OutScaling=2^-10
  Baroreflex : Subsystem
  Bias1 : Bias  Bias=-1
  Constant : Constant  Value=0.8  OutDataType=fixdt(1, 16)  OutScaling=2^0
  Constant1 : Constant  Value=1.66  OutDataType=fixdt(1, 16)  OutScaling=2^0
  Constant2 : Constant  OutDataType=fixdt(1, 16)  OutScaling=2^0
  Constant3 : Constant  OutDataType=fixdt(1, 16)  OutScaling=2^0
  Constant4 : Constant  OutDataType=fixdt(1, 16)  OutScaling=2^0
  Demux2 : Demux  Outputs=3
  Divide1 : Product  Inputs=/*  OutDataType=fixdt(1, 16)  OutScaling=2^-10
  Divide2 : Product  Inputs=**  OutDataType=fixdt(1, 16)  OutScaling=2^-10
  Divide3 : Product  Inputs=*//  OutDataType=fixdt(1, 16)  OutScaling=2^-10
  Divide4 : Product  Inputs=**/  OutDataType=fixdt(1, 16)  OutScaling=2^-10
  Divide8 : Product  Inputs=**/  OutDataType=fixdt(1, 16)  OutScaling=2^-10
  Gain1 : Gain  Gain=1.7  ParameterDataType=fixdt(1, 16)  ParameterScaling=2^0  OutDataType=fixdt(1, 16)  OutScaling=2^0
  Hold1 : ZeroOrderHold  SampleTime=10
  InvSig : Subsystem
  InvSig1 : Subsystem
  Mux1 : Mux  Inputs=2
  Mux3 : Mux  Inputs=2
  Product{,1..3,6} (5 alike) : Product  OutDataType=fixdt(1, 16)  OutScaling=2^0  RndMeth=Zero
  Saturation1 : Saturate  UpperLimit=1  LowerLimit=0  OutDataType=fixdt(1, 16)  OutScaling=2^0
  Scope1 : Scope
      settings: YMin=-13  YMax=1  SaveName=ScopeData18
  Scope2 : Scope
      settings: YMin=90  YMax=230  SaveName=ScopeData21
  Scope3 : Scope
      settings: YMin=90  YMax=230  SaveName=ScopeData22
  Mod_Cardiac_Symp : Outport
  Mod_Arterial_Symp : Outport  Port=2
  Mod_Cardiac_Vagal : Outport  Port=3
  P0 : Outport  Port=4
  wires:
  BP_err/1 -> Add4/2
  HR_err/1 -> Add3/1
  HR_in/1 -> Add2/2, Divide4/1
  Constant1/1 -> Add2/1
  Add3/1 -> Divide1/2
  Add1/1 -> Divide1/1
  Gain1/1 -> Add3/3
  Add2/1 -> Gain1/1
  [Beta_H] -> Add3/2, Add1/2
  [V_H] -> Add1/1
  BP_in/1 -> InvSig1/2(BP_in), Divide8/3, InvSig/2(BP_in), Baroreflex/1(BP_in)
  InvSig/1(P0) -> Mux3/1, Product/1
  Divide2/1 -> Divide8/2
  Divide8/1 -> Divide3/2, Abs/1
  Add4/1 -> Divide8/1
  Ca/1 -> Divide4/3, Divide2/2
  Ra/1 -> Divide2/1
  Divide4/1 -> Add4/1
  InvSig1/1(P0) -> Mux3/2, Product1/2
  Mux3/1 -> Scope2/1
  Mux1/1 -> Scope1/1
  Abs/1 -> Bias1/1
  Bias1/1 -> Divide3/1
  [Alpha] -> Divide3/3
  Divide3/1 -> Saturation1/1
  Constant3/1 -> Add5/2
  Add5/1 -> InvSig1/1(Input), Mux1/2
  Saturation1/1 -> Add5/1
  Add6/1 -> Hold1/1
  Baroreflex/1(Tp) -> Product3/2, Add7/2
  Constant2/1 -> Add7/1
  [AlphaSig] -> InvSig1/3(AlphaSig)
  [AlphaSig] -> InvSig/3(AlphaSig)
  [AlphaSig] -> Baroreflex/3(Alpha_Sig)
  Add7/1 -> Product2/2, Product6/2, Scope3/1
  Product/1 -> Add6/1
  ANS/1 -> Demux2/1
  Demux2/2 -> [Alpha]
  Divide1/1 -> Abs1/1
  Demux2/3 -> [Beta_H]
  Demux2/1 -> [V_H]
  Abs1/1 -> Mux1/1, InvSig/1(Input)
  Constant/1 -> Product/2, Add/1
  Product1/1 -> Add6/2
  Add/1 -> Product1/1
  Constant4/1 -> Add/2
  StrokeVolume/1 -> Divide4/2
  Alpha_Sig/1 -> [AlphaSig]
  Hold1/1 -> P0/1, Baroreflex/2(P0)
  [Beta_H] -> Product6/1
  Product6/1 -> Mod_Cardiac_Symp/1
  [Alpha] -> Product2/1
  Product2/1 -> Mod_Arterial_Symp/1
  [V_H] -> Product3/1
  Product3/1 -> Mod_Cardiac_Vagal/1

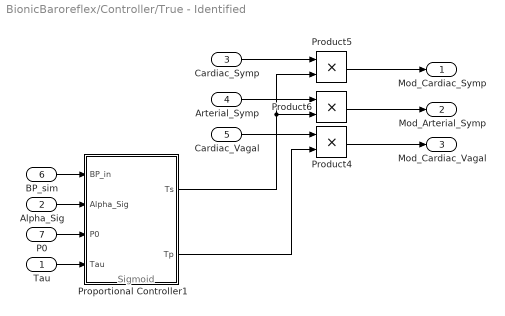
== system BionicBaroreflex/Controller/True - Identified ==
  note: Sigmoid
  Tau : Inport
  Alpha_Sig : Inport  Port=2
  Cardiac_Symp : Inport  Port=3
  Arterial_Symp : Inport  Port=4
  Cardiac_Vagal : Inport  Port=5
  BP_sim : Inport  Port=6
  P0 : Inport  Port=7
  Product4 : Product  OutDataType=fixdt(1, 16)  OutScaling=2^0  RndMeth=Zero
  Product5 : Product  OutDataType=fixdt(1, 16)  OutScaling=2^0  RndMeth=Zero
  Product6 : Product  OutDataType=fixdt(1, 16)  OutScaling=2^0  RndMeth=Zero
  Proportional Controller1 : Subsystem
  Mod_Cardiac_Symp : Outport
  Mod_Arterial_Symp : Outport  Port=2
  Mod_Cardiac_Vagal : Outport  Port=3
  wires:
  Proportional Controller1/2(Tp) -> Product4/2
  Proportional Controller1/1(Ts) -> Product6/2, Product5/2
  Cardiac_Symp/1 -> Product5/1
  Product5/1 -> Mod_Cardiac_Symp/1
  Arterial_Symp/1 -> Product6/1
  Product6/1 -> Mod_Arterial_Symp/1
  Cardiac_Vagal/1 -> Product4/1
  Product4/1 -> Mod_Cardiac_Vagal/1
  BP_sim/1 -> Proportional Controller1/1(BP_in)
  Alpha_Sig/1 -> Proportional Controller1/2(Alpha_Sig)
  P0/1 -> Proportional Controller1/3(P0)
  Tau/1 -> Proportional Controller1/4(Tau)

== system BionicBaroreflex/Data_Import/Artificial CV ==
  Add10 : Sum  OutDataType=fixdt(1, 16)  OutScaling=2^-10
  Add9 : Sum  OutDataType=fixdt(1, 16)  OutScaling=2^-10
  Memory6 : Memory  X0=1.17  InheritSampleTime=on  LinearizeAsDelay=on
  Saturation5 : Saturate  UpperLimit=2.24  LowerLimit=0.58  OutDataType=fixdt(1, 16)  OutScaling=2^0
  Step : Step  Time=500  After=0.5  SampleTime=0
  Uniform Random Number6 : UniformRandomNumber  Minimum=-0.025  Maximum=0.025  SampleTime=10
  Artificial CardiacVagal : Outport
  wires:
  Add9/1 -> Saturation5/1
  Uniform Random Number6/1 -> Add9/2
  Memory6/1 -> Add9/1
  Saturation5/1 -> Memory6/1, Add10/2
  Step/1 -> Add10/1
  Add10/1 -> Artificial CardiacVagal/1

== system BionicBaroreflex/Data_Import/Subsystem ==
  Add1 : Sum  OutDataType=fixdt(1, 16)  OutScaling=2^-10
  Add3 : Sum  OutDataType=fixdt(1, 16)  OutScaling=2^-10
  Memory2 : Memory  X0=0.84  InheritSampleTime=on  LinearizeAsDelay=on
  Saturation3 : Saturate  UpperLimit=1.68  LowerLimit=0.42  OutDataType=fixdt(1, 16)  OutScaling=2^0
  Step : Step  Time=500  After=0.5  SampleTime=0
  Uniform Random Number5 : UniformRandomNumber  Minimum=-0.025  Maximum=0.025  Seed=1  SampleTime=10
  Artificial CardiacSymp : Outport
  wires:
  Memory2/1 -> Add1/1
  Uniform Random Number5/1 -> Add1/2
  Add1/1 -> Saturation3/1
  Saturation3/1 -> Memory2/1, Add3/2
  Step/1 -> Add3/1
  Add3/1 -> Artificial CardiacSymp/1

== system BionicBaroreflex/Data_Import/Subsystem1 ==
  Add1 : Sum  OutDataType=fixdt(1, 16)  OutScaling=2^-10
  Add2 : Sum  OutDataType=fixdt(1, 16)  OutScaling=2^-10
  Memory1 : Memory  X0=1.3  InheritSampleTime=on  LinearizeAsDelay=on
  Saturation : Saturate  UpperLimit=2.6  LowerLimit=0.65  OutDataType=fixdt(1, 16)  OutScaling=2^0
  Step : Step  Time=500  After=0.5  SampleTime=0
  Uniform Random Number3 : UniformRandomNumber  Minimum=-0.025  Maximum=0.025  Seed=2  SampleTime=10
  Artificial ArterialSymp : Outport
  wires:
  Memory1/1 -> Add2/1
  Uniform Random Number3/1 -> Add2/2
  Add2/1 -> Saturation/1
  Saturation/1 -> Memory1/1, Add1/2
  Step/1 -> Add1/1
  Add1/1 -> Artificial ArterialSymp/1

== system BionicBaroreflex/Data_Import/Subsystem2 ==
  Add5 : Sum  OutDataType=fixdt(1, 16)  OutScaling=2^-10
  Memory5 : Memory  X0=1.3
  Saturation4 : Saturate  UpperLimit=100  LowerLimit=25  OutDataType=fixdt(1, 16)  OutScaling=2^0
  Uniform Random Number4 : UniformRandomNumber  Minimum=-0.1  Maximum=0.1  SampleTime=500
  Artificial SV : Outport
  wires:
  Memory5/1 -> Add5/1
  Uniform Random Number4/1 -> Add5/2
  Add5/1 -> Saturation4/1
  Saturation4/1 -> Memory5/1, Artificial SV/1

== system BionicBaroreflex/Data_Import/Subsystem3 ==
  Add1 : Sum  OutDataType=fixdt(1, 16)  OutScaling=2^-10
  Add4 : Sum  OutDataType=fixdt(1, 16)  OutScaling=2^-10
  Memory4 : Memory  X0=100  InheritSampleTime=on  LinearizeAsDelay=on
  Saturation2 : Saturate  UpperLimit=200  LowerLimit=50  OutDataType=fixdt(1, 16)  OutScaling=2^0
  Step : Step  Time=500  After=30  SampleTime=0
  Uniform Random Number1 : UniformRandomNumber  Minimum=-5  Maximum=5  SampleTime=20
  Artificial P0 : Outport
  wires:
  Memory4/1 -> Add4/1
  Uniform Random Number1/1 -> Add4/2
  Add4/1 -> Saturation2/1
  Saturation2/1 -> Memory4/1, Add1/2
  Step/1 -> Add1/1
  Add1/1 -> Artificial P0/1

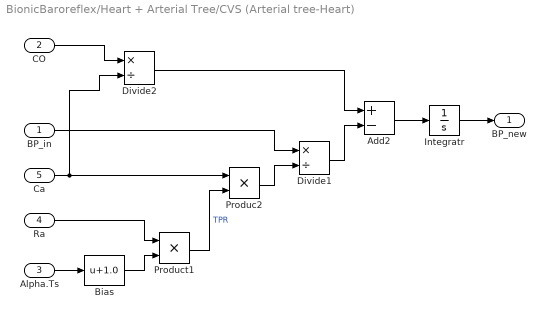
== system BionicBaroreflex/Heart + Arterial Tree/CVS (Arterial tree-Heart) ==
  BP_in : Inport
  CO : Inport  Port=2
  Alpha.Ts : Inport  Port=3
  Ra : Inport  Port=4
  Ca : Inport  Port=5
  Add2 : Sum  Inputs=+-  OutDataType=fixdt(1, 16)  OutScaling=2^-10
  Bias : Bias  Bias=1.0
  Divide1 : Product  Inputs=*/  OutDataType=fixdt(1, 16)  OutScaling=2^-10
  Divide2 : Product  Inputs=*/  OutDataType=fixdt(1, 16)  OutScaling=2^-10
  Integratr : Integrator  InitialCondition=100
  Produc2 : Product  OutDataType=fixdt(1, 16)  OutScaling=2^0  RndMeth=Zero
  Product1 : Product  OutDataType=fixdt(1, 16)  OutScaling=2^0  RndMeth=Zero
  BP_new : Outport
  wires:
  Add2/1 -> Integratr/1
  BP_in/1 -> Divide1/1
  Integratr/1 -> BP_new/1
  Divide2/1 -> Add2/1
  CO/1 -> Divide2/1
  Product1/1 -> Produc2/2  "TPR"
  Bias/1 -> Product1/2
  Ra/1 -> Product1/1
  Alpha.Ts/1 -> Bias/1
  Divide1/1 -> Add2/2
  Produc2/1 -> Divide1/2
  Ca/1 -> Produc2/1, Divide2/2

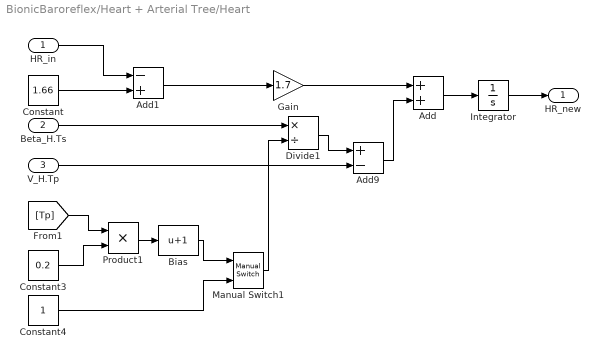
== system BionicBaroreflex/Heart + Arterial Tree/Heart ==
  HR_in : Inport
  Beta_H.Ts : Inport  Port=2
  V_H.Tp : Inport  Port=3
  Add : Sum  OutDataType=fixdt(1, 16)  OutScaling=2^-10
  Add1 : Sum  Inputs=-+  OutDataType=fixdt(1, 16)  OutScaling=2^-10
  Add9 : Sum  Inputs=+-  OutDataType=fixdt(1, 16)  OutScaling=2^-10
  Bias : Bias  Bias=1
  Constant : Constant  Value=1.66  OutDataType=fixdt(1, 16)  OutScaling=2^0
  Constant3 : Constant  Value=0.2  OutDataType=fixdt(1, 16)  OutScaling=2^0
  Constant4 : Constant  OutDataType=fixdt(1, 16)  OutScaling=2^0
  Divide1 : Product  Inputs=*/  OutDataType=fixdt(1, 16)  OutScaling=2^-10
  Gain : Gain  Gain=1.7  ParameterDataType=fixdt(1, 16)  ParameterScaling=2^0  OutDataType=fixdt(1, 16)  OutScaling=2^0
  Integrator : Integrator  InitialCondition=1.66
  Manual Switch1 : simulink/Signal Routing/Manual Switch  SystemSampleTime=-1  sw=0  action=0  varsize=off
  Product1 : Product  OutDataType=fixdt(1, 16)  OutScaling=2^0  RndMeth=Zero
  HR_new : Outport
  wires:
  Constant/1 -> Add1/2
  Add1/1 -> Gain/1
  Gain/1 -> Add/1
  HR_in/1 -> Add1/1
  Add/1 -> Integrator/1
  Add9/1 -> Add/2
  [Tp] -> Product1/1
  Constant3/1 -> Product1/2
  Product1/1 -> Bias/1
  Beta_H.Ts/1 -> Divide1/1
  Divide1/1 -> Add9/1
  V_H.Tp/1 -> Add9/2
  Bias/1 -> Manual Switch1/1
  Manual Switch1/1 -> Divide1/2
  Constant4/1 -> Manual Switch1/2
  Integrator/1 -> HR_new/1

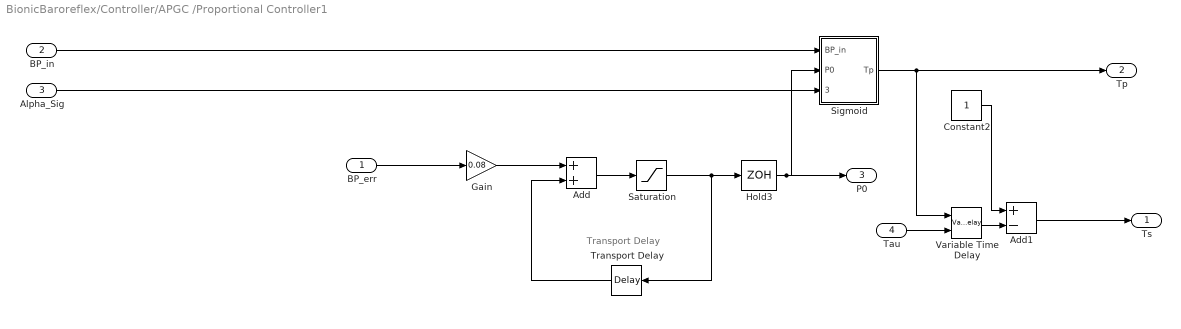
== system BionicBaroreflex/Controller/APGC /Proportional Controller1 ==
  note: Transport Delay
  BP_err : Inport
  BP_in : Inport  Port=2
  Alpha_Sig : Inport  Port=3
  Tau : Inport  Port=4
  Add : Sum  OutDataType=fixdt(1, 16)  OutScaling=2^-10
  Add1 : Sum  Inputs=+-  OutDataType=fixdt(1, 16)  OutScaling=2^-10
  Constant2 : Constant  OutDataType=fixdt(1, 16)  OutScaling=2^0
  Gain : Gain  Gain=0.08  ParameterDataType=fixdt(1, 16)  ParameterScaling=2^0  OutDataType=fixdt(1, 16)  OutScaling=2^0
  Hold3 : ZeroOrderHold  SampleTime=30
  Saturation : Saturate  UpperLimit=200  LowerLimit=0  OutDataType=fixdt(1, 16)  OutScaling=2^0
  Sigmoid : Subsystem
  Transport Delay : TransportDelay  InitialOutput=100
  Variable Time Delay : VariableTransportDelay  MaximumDelay=10
  Ts : Outport
  Tp : Outport  Port=2
  P0 : Outport  Port=3
  wires:
  Tau/1 -> Variable Time Delay/2
  Variable Time Delay/1 -> Add1/2
  Saturation/1 -> Hold3/1, Transport Delay/1
  Add/1 -> Saturation/1
  BP_in/1 -> Sigmoid/1(BP_in)
  Sigmoid/1(Tp) -> Variable Time Delay/1, Tp/1
  Constant2/1 -> Add1/1
  Alpha_Sig/1 -> Sigmoid/3(Alpha_Sig)
  Add1/1 -> Ts/1
  Hold3/1 -> P0/1, Sigmoid/2(P0)
  Transport Delay/1 -> Add/2
  BP_err/1 -> Gain/1
  Gain/1 -> Add/1

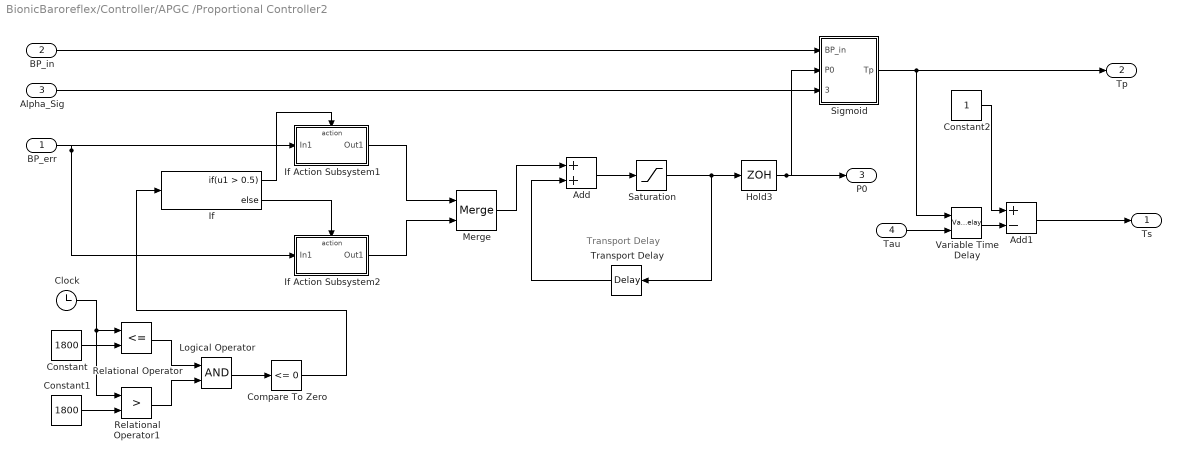
== system BionicBaroreflex/Controller/APGC /Proportional Controller2 ==
  note: Transport Delay
  BP_err : Inport
  BP_in : Inport  Port=2
  Alpha_Sig : Inport  Port=3
  Tau : Inport  Port=4
  Add : Sum  OutDataType=fixdt(1, 16)  OutScaling=2^-10
  Add1 : Sum  Inputs=+-  OutDataType=fixdt(1, 16)  OutScaling=2^-10
  Clock : Clock
      settings: Decimation=10
  Compare To Zero : simulink/Logic and Bit Operations/Compare To Zero  SystemSampleTime=-1  relop=<=  LogicOutDataTypeMode=uint8  ZeroCross=off
  Constant : Constant  Value=1800  OutDataType=fixdt(1, 16)  OutScaling=2^0
  Constant1 : Constant  Value=1800  OutDataType=fixdt(1, 16)  OutScaling=2^0
  Constant2 : Constant  OutDataType=fixdt(1, 16)  OutScaling=2^0
  Hold3 : ZeroOrderHold  SampleTime=30
  If : If  IfExpression=u1 > 0.5
  If Action Subsystem1 : Subsystem  TreatAsAtomicUnit=on
  If Action Subsystem2 : Subsystem  TreatAsAtomicUnit=on
  Logical Operator : Logic  AllPortsSameDT=off  OutDataTypeMode=boolean  LogicDataType=fixdt(0, 8)  OutDataTypeStr=boolean
  Merge : Merge
  Relational Operator : RelationalOperator  Operator=<=  LogicOutDataTypeMode=boolean  LogicDataType=fixdt(0, 8)  OutDataTypeStr=boolean
  Relational Operator1 : RelationalOperator  Operator=>  LogicOutDataTypeMode=boolean  LogicDataType=fixdt(0, 8)  OutDataTypeStr=boolean
  Saturation : Saturate  UpperLimit=200  LowerLimit=0  OutDataType=fixdt(1, 16)  OutScaling=2^0
  Sigmoid : Subsystem
  Transport Delay : TransportDelay  InitialOutput=100
  Variable Time Delay : VariableTransportDelay  MaximumDelay=10
  Ts : Outport
  Tp : Outport  Port=2
  P0 : Outport  Port=3
  wires:
  Transport Delay/1 -> Add/2
  Hold3/1 -> Sigmoid/2(P0), P0/1
  Add1/1 -> Ts/1
  Alpha_Sig/1 -> Sigmoid/3(Alpha_Sig)
  Constant2/1 -> Add1/1
  Sigmoid/1(Tp) -> Tp/1, Variable Time Delay/1
  BP_in/1 -> Sigmoid/1(BP_in)
  Add/1 -> Saturation/1
  Saturation/1 -> Transport Delay/1, Hold3/1
  Clock/1 -> Relational Operator/1, Relational Operator1/1
  Constant/1 -> Relational Operator/2
  Compare To Zero/1 -> If/1
  BP_err/1 -> If Action Subsystem1/1(In1), If Action Subsystem2/1(In1)
  If/1 -> If Action Subsystem1/Action
  If/2 -> If Action Subsystem2/Action
  If Action Subsystem1/1(Out1) -> Merge/1
  Merge/1 -> Add/1
  If Action Subsystem2/1(Out1) -> Merge/2
  Constant1/1 -> Relational Operator1/2
  Relational Operator/1 -> Logical Operator/1
  Relational Operator1/1 -> Logical Operator/2
  Logical Operator/1 -> Compare To Zero/1
  Variable Time Delay/1 -> Add1/2
  Tau/1 -> Variable Time Delay/2

== system BionicBaroreflex/Controller/Controller/Baroreflex ==
  BP_in : Inport
  P0 : Inport  Port=2
  Alpha_Sig : Inport  Port=3
  Add4 : Sum  Inputs=+-  OutDataType=fixdt(1, 16)  OutScaling=2^-10
  Fcn : Fcn  Expr=1/(1+exp(u))
  Gain1 : Gain  Gain=-1  ParameterDataType=fixdt(1, 16)  ParameterScaling=2^0  OutDataType=fixdt(1, 16)  OutScaling=2^0
  Product4 : Product  OutDataType=fixdt(1, 16)  OutScaling=2^0  RndMeth=Zero
  Tp : Outport
  wires:
  Add4/1 -> Product4/1
  Gain1/1 -> Fcn/1
  Product4/1 -> Gain1/1
  BP_in/1 -> Add4/1
  Fcn/1 -> Tp/1
  Alpha_Sig/1 -> Product4/2
  P0/1 -> Add4/2

== system BionicBaroreflex/Controller/Controller/InvSig ==
  Input : Inport
  BP_in : Inport  Port=2
  AlphaSig : Inport  Port=3
  Add4 : Sum  OutDataType=fixdt(1, 16)  OutScaling=2^-10
  Bias2 : Bias  Bias=-1
  Divide2 : Product  Inputs=*/  OutDataType=fixdt(1, 16)  OutScaling=2^-10
  Math Function : Math  Operator=log  OutDataType=fixdt(1, 16)  OutScaling=2^0  SaturateOnIntegerOverflow=on
  Math Function1 : Math  Operator=reciprocal  OutDataType=fixdt(1, 16)  OutScaling=2^0  SaturateOnIntegerOverflow=on
  Saturation : Saturate  UpperLimit=200  LowerLimit=0  OutDataType=fixdt(1, 16)  OutScaling=2^0
  Saturation1 : Saturate  UpperLimit=0.99  LowerLimit=0.01  OutDataType=fixdt(1, 16)  OutScaling=2^0
  Scope1 : Scope
      settings: YMin=5  YMax=100  SaveName=ScopeData19
  Scope2 : Scope
      settings: YMin=95  YMax=185  SaveName=ScopeData20
  P0 : Outport
  wires:
  Add4/1 -> Saturation/1
  Math Function/1 -> Divide2/1
  Divide2/1 -> Add4/1
  BP_in/1 -> Add4/2
  AlphaSig/1 -> Divide2/2
  Math Function1/1 -> Bias2/1
  Input/1 -> Saturation1/1
  Bias2/1 -> Math Function/1, Scope1/1
  Saturation1/1 -> Math Function1/1
  Saturation/1 -> P0/1, Scope2/1

== system BionicBaroreflex/Controller/Controller/InvSig1 ==
  Input : Inport
  BP_in : Inport  Port=2
  AlphaSig : Inport  Port=3
  Add4 : Sum  OutDataType=fixdt(1, 16)  OutScaling=2^-10
  Bias2 : Bias  Bias=-1
  Divide2 : Product  Inputs=*/  OutDataType=fixdt(1, 16)  OutScaling=2^-10
  Math Function : Math  Operator=log  OutDataType=fixdt(1, 16)  OutScaling=2^0  SaturateOnIntegerOverflow=on
  Math Function1 : Math  Operator=reciprocal  OutDataType=fixdt(1, 16)  OutScaling=2^0  SaturateOnIntegerOverflow=on
  Saturation : Saturate  UpperLimit=200  LowerLimit=0  OutDataType=fixdt(1, 16)  OutScaling=2^0
  Saturation1 : Saturate  UpperLimit=0.99  LowerLimit=0.01  OutDataType=fixdt(1, 16)  OutScaling=2^0
  Scope1 : Scope
      settings: YMin=5  YMax=100  SaveName=ScopeData16
  Scope2 : Scope
      settings: YMin=95  YMax=185  SaveName=ScopeData17
  P0 : Outport
  wires:
  Saturation1/1 -> Math Function1/1
  Bias2/1 -> Scope1/1, Math Function/1
  Input/1 -> Saturation1/1
  Math Function1/1 -> Bias2/1
  AlphaSig/1 -> Divide2/2
  BP_in/1 -> Add4/2
  Divide2/1 -> Add4/1
  Math Function/1 -> Divide2/1
  Add4/1 -> Saturation/1
  Saturation/1 -> Scope2/1, P0/1

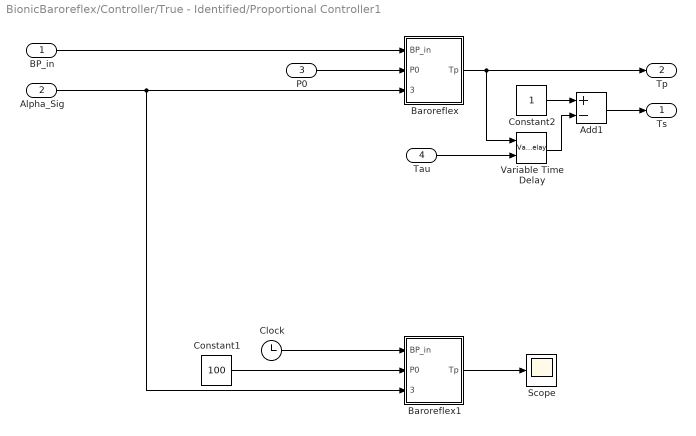
== system BionicBaroreflex/Controller/True - Identified/Proportional Controller1 ==
  BP_in : Inport
  Alpha_Sig : Inport  Port=2
  P0 : Inport  Port=3
  Tau : Inport  Port=4
  Add1 : Sum  Inputs=+-  OutDataType=fixdt(1, 16)  OutScaling=2^-10
  Baroreflex : Subsystem
  Baroreflex1 : Subsystem
  Clock : Clock
      settings: Decimation=10
  Constant1 : Constant  Value=100  OutDataType=fixdt(1, 16)  OutScaling=2^0
  Constant2 : Constant  OutDataType=fixdt(1, 16)  OutScaling=2^0
  Scope : Scope
      settings: YMin=0.0754666  YMax=0.0834104  SaveName=ScopeData3
  Variable Time Delay : VariableTransportDelay  MaximumDelay=10
  Ts : Outport
  Tp : Outport  Port=2
  wires:
  BP_in/1 -> Baroreflex/1(BP_in)
  Baroreflex/1(Tp) -> Tp/1, Variable Time Delay/1
  Constant2/1 -> Add1/1
  Alpha_Sig/1 -> Baroreflex1/3(Alpha_Sig), Baroreflex/3(Alpha_Sig)
  Add1/1 -> Ts/1
  P0/1 -> Baroreflex/2(P0)
  Variable Time Delay/1 -> Add1/2
  Tau/1 -> Variable Time Delay/2
  Clock/1 -> Baroreflex1/1(BP_in)
  Baroreflex1/1(Tp) -> Scope/1
  Constant1/1 -> Baroreflex1/2(P0)

== system BionicBaroreflex/Controller/APGC /Proportional Controller1/Sigmoid ==
  BP_in : Inport
  P0 : Inport  Port=2
  Alpha_Sig : Inport  Port=3
  Add4 : Sum  Inputs=+-  OutDataType=fixdt(1, 16)  OutScaling=2^-10
  Fcn : Fcn  Expr=1/(1+exp(u))
  Gain1 : Gain  Gain=-1  ParameterDataType=fixdt(1, 16)  ParameterScaling=2^0  OutDataType=fixdt(1, 16)  OutScaling=2^0
  Product4 : Product  OutDataType=fixdt(1, 16)  OutScaling=2^0  RndMeth=Zero
  Tp : Outport
  wires:
  Add4/1 -> Product4/1
  Gain1/1 -> Fcn/1
  Product4/1 -> Gain1/1
  BP_in/1 -> Add4/1
  Fcn/1 -> Tp/1
  Alpha_Sig/1 -> Product4/2
  P0/1 -> Add4/2

== system BionicBaroreflex/Controller/APGC /Proportional Controller2/If Action Subsystem1 ==
  In1 : Inport  OutDataType=fixdt(1, 16)  OutScaling=2^0
  Action Port : ActionPort  PropagateVarSize=During execution  ActionType=then
  Gain : Gain  Gain=0.08  ParameterDataType=fixdt(1, 16)  ParameterScaling=2^0  OutDataType=fixdt(1, 16)  OutScaling=2^0
  Out1 : Outport  OutDataType=fixdt(1, 16)  OutScaling=2^0
  wires:
  Gain/1 -> Out1/1
  In1/1 -> Gain/1

== system BionicBaroreflex/Controller/APGC /Proportional Controller2/If Action Subsystem2 ==
  In1 : Inport  OutDataType=fixdt(1, 16)  OutScaling=2^0
  Action Port : ActionPort  PropagateVarSize=During execution  ActionType=else
  Gain : Gain  Gain=-0.08  ParameterDataType=fixdt(1, 16)  ParameterScaling=2^0  OutDataType=fixdt(1, 16)  OutScaling=2^0
  Out1 : Outport  OutDataType=fixdt(1, 16)  OutScaling=2^0
  wires:
  In1/1 -> Gain/1
  Gain/1 -> Out1/1

== system BionicBaroreflex/Controller/APGC /Proportional Controller2/Sigmoid ==
  BP_in : Inport
  P0 : Inport  Port=2
  Alpha_Sig : Inport  Port=3
  Add4 : Sum  Inputs=+-  OutDataType=fixdt(1, 16)  OutScaling=2^-10
  Fcn : Fcn  Expr=1/(1+exp(u))
  Gain1 : Gain  Gain=-1  ParameterDataType=fixdt(1, 16)  ParameterScaling=2^0  OutDataType=fixdt(1, 16)  OutScaling=2^0
  Product4 : Product  OutDataType=fixdt(1, 16)  OutScaling=2^0  RndMeth=Zero
  Tp : Outport
  wires:
  P0/1 -> Add4/2
  Alpha_Sig/1 -> Product4/2
  Fcn/1 -> Tp/1
  BP_in/1 -> Add4/1
  Product4/1 -> Gain1/1
  Gain1/1 -> Fcn/1
  Add4/1 -> Product4/1

== system BionicBaroreflex/Controller/True - Identified/Proportional Controller1/Baroreflex ==
  BP_in : Inport
  P0 : Inport  Port=2
  Alpha_Sig : Inport  Port=3
  Add4 : Sum  Inputs=+-  OutDataType=fixdt(1, 16)  OutScaling=2^-10
  Fcn : Fcn  Expr=1/(1+exp(u))
  Gain1 : Gain  Gain=-1  ParameterDataType=fixdt(1, 16)  ParameterScaling=2^0  OutDataType=fixdt(1, 16)  OutScaling=2^0
  Product4 : Product  OutDataType=fixdt(1, 16)  OutScaling=2^0  RndMeth=Zero
  Tp : Outport
  wires:
  Add4/1 -> Product4/1
  Gain1/1 -> Fcn/1
  Product4/1 -> Gain1/1
  BP_in/1 -> Add4/1
  Fcn/1 -> Tp/1
  Alpha_Sig/1 -> Product4/2
  P0/1 -> Add4/2

== system BionicBaroreflex/Controller/True - Identified/Proportional Controller1/Baroreflex1 ==
  BP_in : Inport
  P0 : Inport  Port=2
  Alpha_Sig : Inport  Port=3
  Add4 : Sum  Inputs=+-  OutDataType=fixdt(1, 16)  OutScaling=2^-10
  Fcn : Fcn  Expr=1/(1+exp(u))
  Gain1 : Gain  Gain=-1  ParameterDataType=fixdt(1, 16)  ParameterScaling=2^0  OutDataType=fixdt(1, 16)  OutScaling=2^0
  Product4 : Product  OutDataType=fixdt(1, 16)  OutScaling=2^0  RndMeth=Zero
  Tp : Outport
  wires:
  P0/1 -> Add4/2
  Alpha_Sig/1 -> Product4/2
  Fcn/1 -> Tp/1
  BP_in/1 -> Add4/1
  Product4/1 -> Gain1/1
  Gain1/1 -> Fcn/1
  Add4/1 -> Product4/1
